simulink model "Parallel_HEV"  (R2019b)
settings: Solver=VariableStepAuto  StartTime=0.0  StopTime=1061  RelTol=1e-3
libraries: qss_tb_library x8
settings Model: Creator=badk  LastModifiedBy=murugan

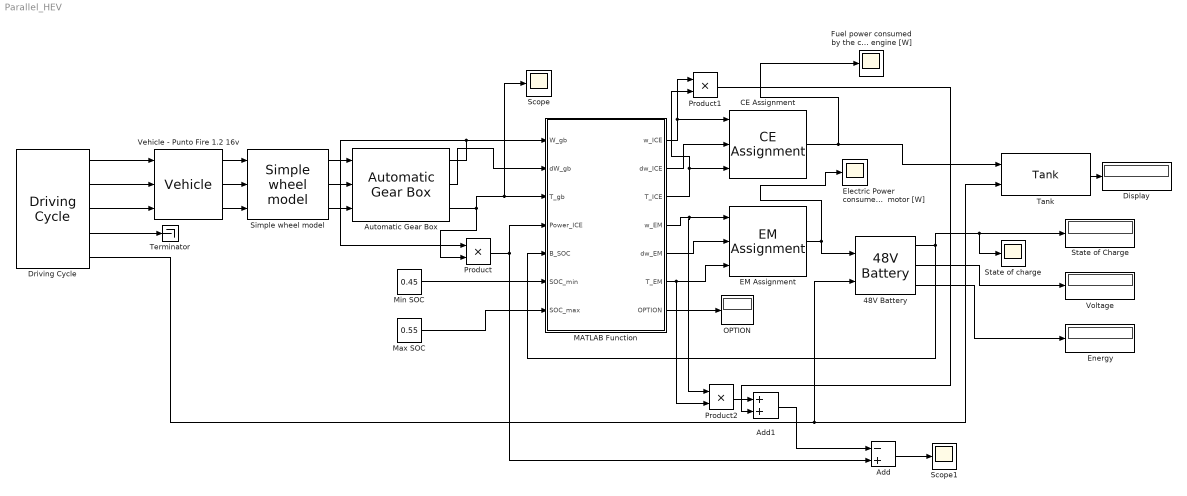
== system Parallel_HEV ==
  48V Battery : qss_tb_library/Energy Buffer/48V Battery  Tag=battery  cell_series=70  cell_parallel=5  Q_BT_IC_rel=49
  Add : Sum  Inputs=-+
  Add1 : Sum
  Automatic Gear Box : qss_tb_library/Gear System/Automatic Gear Box  Tag=transmission  nog=5  i=[3.909 2.158 2.158 1.121 0.921]  i_diff=4.071  gearon=[10 25 40 70]  gearoff=[2 15 30 50]  d=0.5842  e_GT=0.98  P_GT0=300  w_wheel_min=1
  CE Assignment : qss_tb_library/Energy Converter/CE Assignment  Tag=combustion engine  engine_type=Gasoline  P_ice=35  ENABLE_FUEL_CUTOFF=off
  Display : Display
  Driving Cycle : qss_tb_library/Driving Cycle/Driving Cycle  Tag=cycle  cyclename1=customcity  stepsize=1  autostop=on
  EM Assignment : qss_tb_library/Energy Converter/EM Assignment  P_em=25
  Electric Power consumed by the  motor [W] : Scope
  Energy : Display
  Fuel power consumed by the combustion engine [W] : Scope
  MATLAB Function : MATLAB Function  TreatAsAtomicUnit=on
  Max SOC : Constant  Value=0.55
  Min SOC : Constant  Value=0.45
  OPTION : Display
  Product : Product
  Product1 : Product
  Product2 : Product
  Scope : Scope
  Scope1 : Scope
  Simple wheel model : qss_tb_library/Vehicle/Simple wheel model  Tag=simple transmission  d_wheel=0.5842
  State of Charge : Display
  State of charge : Scope
  Tank : qss_tb_library/Energy Source/Tank  Tag=tank  fuel=Gasoline  flag_cold_start=on
  Terminator : Terminator
  Vehicle - Punto Fire 1.2 16v : qss_tb_library/Vehicle/Vehicle  Tag=vehicle  m_f=921+69.5  A_f=(1.48*1.66)  cw=0.31  mu=0.012  k_inertia=4
  Voltage : Display
  wires:
  Vehicle - Punto Fire 1.2 16v/1 -> Simple wheel model/1
  Vehicle - Punto Fire 1.2 16v/2 -> Simple wheel model/2
  Vehicle - Punto Fire 1.2 16v/3 -> Simple wheel model/3
  Driving Cycle/1 -> Vehicle - Punto Fire 1.2 16v/1
  Driving Cycle/2 -> Vehicle - Punto Fire 1.2 16v/2
  Driving Cycle/3 -> Vehicle - Punto Fire 1.2 16v/3
  Simple wheel model/1 -> Automatic Gear Box/1
  MATLAB Function/1(w_ICE) -> Product1/1, CE Assignment/1
  MATLAB Function/2(dw_ICE) -> CE Assignment/2
  MATLAB Function/3(T_ICE) -> Product1/2, CE Assignment/3
  MATLAB Function/4(w_EM) -> Product2/1, EM Assignment/1
  MATLAB Function/5(dw_EM) -> EM Assignment/2
  MATLAB Function/6(T_EM) -> Product2/2, EM Assignment/3
  EM Assignment/1 -> Electric Power consumed by the  motor [W]/1, 48V Battery/1
  Tank/1 -> Display/1
  CE Assignment/1 -> Fuel power consumed by the combustion engine [W]/1, Tank/1
  Driving Cycle/5 -> 48V Battery/2, Tank/2
  Driving Cycle/4 -> Terminator/1
  Simple wheel model/2 -> Automatic Gear Box/2
  Simple wheel model/3 -> Automatic Gear Box/3
  Automatic Gear Box/1 -> Product/1, MATLAB Function/1(W_gb)
  Automatic Gear Box/2 -> MATLAB Function/2(dW_gb)
  Automatic Gear Box/3 -> MATLAB Function/3(T_gb), Scope/1, Product/2
  Product/1 -> Add/2, MATLAB Function/4(Power_ICE)
  48V Battery/1 -> State of charge/1, State of Charge/1, MATLAB Function/5(B_SOC)
  MATLAB Function/7(OPTION) -> OPTION/1
  48V Battery/2 -> Voltage/1
  48V Battery/3 -> Energy/1
  Min SOC/1 -> MATLAB Function/6(SOC_min)
  Max SOC/1 -> MATLAB Function/7(SOC_max)
  Product2/1 -> Add1/1
  Product1/1 -> Add1/2
  Add1/1 -> Add/1
  Add/1 -> Scope1/1

== matlab function Parallel_HEV/MATLAB Function ==
  data: W_gb input; w_ICE output; dW_gb input; T_gb input; Power_ICE input; B_SOC input; SOC_min input; SOC_max input; dw_ICE output; T_ICE output; w_EM output; dw_EM output; T_EM output; OPTION output
function [w_ICE,dw_ICE,T_ICE,w_EM,dw_EM,T_EM,OPTION] = fcn(W_gb,dW_gb,T_gb,Power_ICE,B_SOC,SOC_min,SOC_max)

%initialize

power_demand = (W_gb*T_gb);
optimum_w = (2500/60)*2*pi;
optimum_T = 100.5;

%High SOC and High power demand (IC engine running & Electrical Motor on)
if B_SOC>SOC_max && Power_ICE>35e3
    
        w_ICE = W_gb;
        dw_ICE = dW_gb;
        T_ICE = T_gb;
        
        w_EM = W_gb;
        dw_EM = dW_gb;
        T_EM = dW_gb;
        
        OPTION = 1;
        
%High SOC and Low power demand (Electrical Motor running & Engine off )
    elseif B_SOC>SOC_max && Power_ICE<35e3
        
        w_ICE = 0;
        dw_ICE = 0;
        T_ICE = 0;   
        
        w_EM = W_gb;
        dw_EM = dW_gb;
        T_EM = T_gb;
        
        OPTION = 2;

%Low SOC and High power demand (Engine running & Battery charging)
    elseif B_SOC<SOC_min && Power_ICE>35e3 %&& T_gb>optimum_T
        
        w_ICE = W_gb;
        dw_ICE = dW_gb;
        T_ICE = T_gb; 
        
        w_EM = 0;
        dw_EM = 0;
        T_EM = 0;
        
        OPTION = 3;
        
elseif B_SOC<SOC_min && T_gb<optimum_T %charging
        
        w_ICE = W_gb;
        dw_ICE = dW_gb;
        T_ICE = optimum_T; %T_gb
        
        w_EM = W_gb;
        dw_EM = dW_gb;
        T_EM = (power_demand-Power_ICE)/W_gb; %-ve tor
        
        OPTION = 4;
        
    %high Power demand (Engine running & Electric assist)
    elseif T_gb>optimum_T
        
        w_ICE = W_gb;
        dw_ICE = dW_gb;
        T_ICE = optimum_T;  %T_gb
        
        w_EM = W_gb;
        dw_EM = dW_gb;
        T_EM = (power_demand-Power_ICE)/W_gb; %+ve torq
        
        OPTION = 5;
        
%Regenerative braking
    elseif Power_ICE<0
        
        w_ICE = 0;
        dw_ICE = 0;
        T_ICE = 0;
        
        w_EM = W_gb;
        dw_EM = dW_gb;
        T_EM = T_gb;
        
        OPTION = 6;
        
elseif B_SOC>=SOC_min && B_SOC<=SOC_max && Power_ICE>0
    
    w_ICE=W_gb;
    T_ICE=0.64*T_gb;
    dw_ICE=dW_gb;   
    
    w_EM=W_gb;
    T_EM=T_gb-T_ICE;
    dw_EM=dW_gb;
    
    OPTION = 7;
    
%Vehicle comes to standstill position        
else
    w_ICE = 0;              %setting parameters to zero
    dw_ICE = 0;
    T_ICE = 0;
    w_EM = 0;
    dw_EM = 0;
    T_EM = 0;

    OPTION = 0;





end



end
